simulink model "QPSK_NDATED_DDPED_R2021"  (R2021b)
settings: Solver=ode45  StartTime=0  StopTime=800*6  RelTol=1e-3  EnableMultiTasking=on
PreLoadFcn:
  | SNR=15;                          % Signal-to-noise ratio
  | T =  0.1;                          % Symbol period
  | Tc = T/10;                       % Carrier period
  | deltaf = (3/360)/T;;         % Frequency error
  | deltaT = 300e-6;             % Timing error
  | Tr = T*(1+deltaT);           % Receiver clock
  | alpha = 0.5;                     % Rolloff factor
  | b3 = [1/6 -1/2  1/2 -1/6];
  | b2 = [1/2 -1    1/2  0];
  | b1 = [1/3  1/2 -1    1/6];
  | b0 = [0    1    0    0];
  | warning off all
undefined symbols (not defined in the file or in its folder): dfilt, gcbh, rcfiltgaincompat
libraries: dspobslib x7, commfilt2 x4, dsparch4 x3, commchan3 x1, commdigbbndpm3 x1, commrandsrc2 x1
settings Model: SimulationMode=accelerator  Creator=professor  LastModifiedBy=14083
settings SolverCC: AlgebraicLoopSolver=TrustRegion
settings DataIOCC: LimitDataPoints=on  SaveFormat=Array  SignalLoggingSaveFormat=ModelDataLogs  ReturnWorkspaceOutputs=off
settings OptimizationCC: ExpressionDepthLimit=2147483647  InitFltsAndDblsToZero=on  LifeSpan=inf
settings DebuggingCC: AlgebraicLoopMsg=none  SaveWithParameterizedLinksMsg=none  UnderspecifiedInitializationDetection=Classic  MergeDetectMultiDrivingBlocksExec=none  SolverPrmCheckMsg=warning  MultiTaskDSMMsg=warning  MultiTaskCondExecSysMsg=none  FcnCallInpInsideContextMsg=warning  StateNameClashWarn=warning  SFUnexpectedBacktrackingDiag=warning  SFNoUnconditionalDefaultTransitionDiag=warning  SFExecutionAtInitializationDiag=none  SFMachineParentedDataDiag=warning  ArithmeticOperatorsInVariantConditions=warning
settings HardwareCC: ProdBitPerPointer=32  ProdBitPerSizeT=32  ProdBitPerPtrDiffT=32  ProdLargestAtomicFloat=None  ProdIntDivRoundTo=Undefined  ProdEndianess=Unspecified  ProdWordSize=32  ProdHWDeviceType=32-bit Generic
settings ModelReferenceCC: PropagateSignalLabelsOutOfModel=off
settings SFSimCC: SimUseLocalCustomCode=off  CustomCodeUndefinedFunction=UseInterfaceOnly
settings RTWCC: RTWUseLocalCustomCode=off
settings CodeAppCC: StateflowObjectComments=on
settings GRTTargetCC: TargetFcnLib=ansi_tfl_tmw.mat  TargetLangStandard=C89/C90 (ANSI)  CombineOutputUpdateFcns=off  GRTInterface=on
settings ConfigComp: CovMetricSettings=dw  CovSaveCumulativeToWorkspaceVar=on  CovSaveSingleToWorkspaceVar=on  CovExternalEMLEnable=off

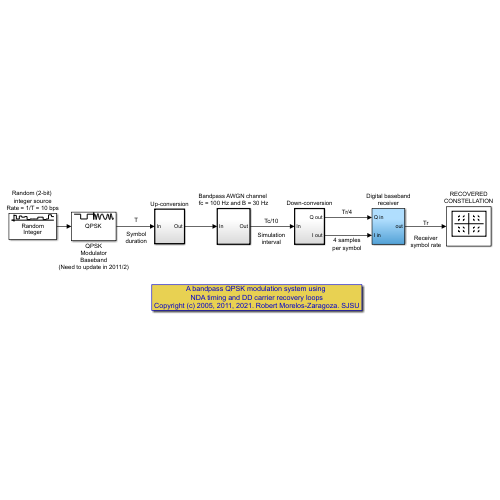
[thumbnail: Simulink's stored preview of the top-level diagram]
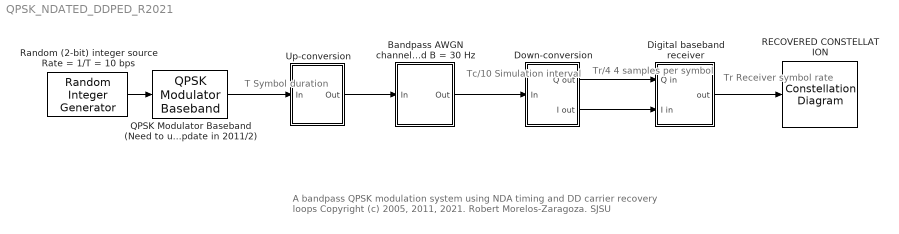
== system QPSK_NDATED_DDPED_R2021 ==
  note: A bandpass QPSK modulation system using
      | NDA timing and DD carrier recovery loops
      | Copyright (c) 2005, 2011, 2021. Robert Morelos-Zaragoza. SJSU
  note: Tc/10
      |
      | Simulation
      | interval
  note: T
      |
      | Symbol
      | duration
  note: Tr/4
      |
      |
      |
      | 4 samples
      | per symbol
  note: Tr
      |
      | Receiver
      | symbol rate
  Bandpass AWGN channel fc = 100 Hz and B = 30 Hz : Subsystem  TreatAsAtomicUnit=on
  Digital baseband receiver : Subsystem
  Down-conversion : Subsystem  TreatAsAtomicUnit=on
  QPSK Modulator Baseband (Need to update in 2011/2) : commdigbbndpm3/QPSK Modulator Baseband  InType=Integer  Enc=Gray  Ph=pi/4  outDtype=double  outWordLen=16  outUDDataType=sfix(16)  outFracLenMode=Best precision  outFracLen=15  outDataTypeStr=double  outLastDataTypeStr=double
  RECOVERED CONSTELLATION : ConstellationDiagram  Tag=ScatterPlot
  Random (2-bit) integer source Rate = 1/T = 10 bps : commrandsrc2/Random Integer Generator  mul=4  seed=15571  Ts=T  frameBased=off  sampPerFrame=1  orient=off  outDataType=double
      settings: SourceProductBaseCode=CM
  Up-conversion : Subsystem  TreatAsAtomicUnit=on
  wires:
  Bandpass AWGN channel fc = 100 Hz and B = 30 Hz/1(Out) -> Down-conversion/1(In)
  Down-conversion/1(Q out) -> Digital baseband receiver/1(Q in)
  Down-conversion/2(I out) -> Digital baseband receiver/2(I in)
  Digital baseband receiver/1(out) -> RECOVERED CONSTELLATION/1
  QPSK Modulator Baseband (Need to update in 2011/2)/1 -> Up-conversion/1(In)
  Random (2-bit) integer source Rate = 1/T = 10 bps/1 -> QPSK Modulator Baseband (Need to update in 2011/2)/1
  Up-conversion/1(Out) -> Bandpass AWGN channel fc = 100 Hz and B = 30 Hz/1(In)

== system QPSK_NDATED_DDPED_R2021/Bandpass AWGN channel fc = 100 Hz and B = 30 Hz ==
  note: Bandpass AWGN channel
      |
      | Robert Morelos-Zaragoza
      | San Jose State University
      | Copyright (c) 2005
  In : Inport
  AWGN Channel : commchan3/AWGN Channel  InputProcessing=Columns as channels (frame based)  seed=13357  noiseMode="Signal to noise ratio  (Eb/No)"  EbNodB=SNR  EsNodB=15  SNRdB=10  bitsPerSym=2  Ps=1  Tsym=T/4  variance=1
  "Channel Hc(f) fc=100, B=30" : dsparch4/Analog Filter Design  method=Chebyshev I  filttype=Bandpass  N=20  Wlo=2*pi*85  Whi=2*pi*115  Rp=0.5  Rs=30
  Tc/10 Simulation interval : ZeroOrderHold  SampleTime=Tc/10
  Out : Outport
  wires:
  "Channel Hc(f) fc=100, B=30"/1 -> Tc/10 Simulation interval/1
  AWGN Channel/1 -> Out/1
  In/1 -> "Channel Hc(f) fc=100, B=30"/1
  Tc/10 Simulation interval/1 -> AWGN Channel/1

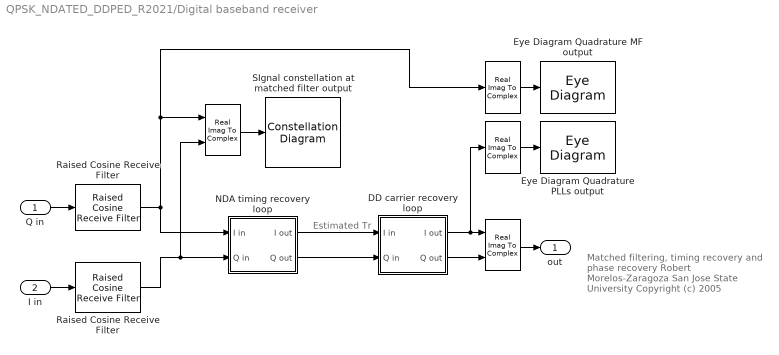
== system QPSK_NDATED_DDPED_R2021/Digital baseband receiver ==
  note: Estimated
      | Tr
  note: Matched filtering, timing recovery
      | and phase recovery
      |
      | Robert Morelos-Zaragoza
      | San Jose State University
      | Copyright (c) 2005
  Q in : Inport
  I in : Inport  Port=2
  " " : RealImagToComplex  Input=Real  SampleTime=Tr/4
  "    " : RealImagToComplex  SampleTime=Tr/4
  "       " : RealImagToComplex  Input=Real  SampleTime=Tr/4
  "           " : RealImagToComplex  SampleTime=Tr
  DD carrier recovery loop : Subsystem
  Eye Diagram Quadrature MF output : EyeDiagram  Tag=EyeDiagram
  Eye Diagram Quadrature PLLs output : EyeDiagram  Tag=EyeDiagram
  NDA timing recovery loop : Subsystem
  Raised Cosine Receive Filter : commfilt2/Raised Cosine Receive Filter  filtType=Square root  R=alpha  filtSpan=2*(4)  N=4  downFactor=1  downOffset=0  filterGain=(1/2)*rcfiltgaincompat(gcbh)  InputProcessing=Columns as channels (frame based)  RateOptions=Enforce single-rate processing  framing=Maintain input frame size  checkCoeff=off  variableName=rcRxFilt  currentFiltSpan=2*(4)  D=4  inputOffset=0  sampMode=Mute  saveAsFlag=0  rateMode=Downsampling  checkGain=User-specified  launchFVT=off  roundingMode=Floor  overflowMode=off  coeffDataTypeStr=Inherit: Same word length as input  coeffMin=[]  coeffMax=[]  coeffLastDataTypeStr=Inherit: Same word length as input  accumDataTypeStr=Inherit: Same as product output  accumLastDataTypeStr=Inherit: Same as product output  outputDataTypeStr=Inherit: Same as accumulator  outputMin=[]  outputMax=[]  outputLastDataTypeStr=Inherit: Same as accumulator
  "Raised Cosine Receive Filter " : commfilt2/Raised Cosine Receive Filter  filtType=Square root  R=alpha  filtSpan=2*(4)  N=4  downFactor=1  downOffset=0  filterGain=(1/2)*rcfiltgaincompat(gcbh)  InputProcessing=Columns as channels (frame based)  RateOptions=Enforce single-rate processing  framing=Maintain input frame size  checkCoeff=off  variableName=rcRxFilt1  currentFiltSpan=2*(4)  D=4  inputOffset=0  sampMode=Mute  saveAsFlag=0  rateMode=Downsampling  checkGain=User-specified  launchFVT=off  roundingMode=Floor  overflowMode=off  coeffDataTypeStr=Inherit: Same word length as input  coeffMin=[]  coeffMax=[]  coeffLastDataTypeStr=Inherit: Same word length as input  accumDataTypeStr=Inherit: Same as product output  accumLastDataTypeStr=Inherit: Same as product output  outputDataTypeStr=Inherit: Same as accumulator  outputMin=[]  outputMax=[]  outputLastDataTypeStr=Inherit: Same as accumulator
  SIgnal constellation at matched filter output : ConstellationDiagram  Tag=ScatterPlot
  out : Outport
  wires:
  Q in/1 -> Raised Cosine Receive Filter/1
  I in/1 -> "Raised Cosine Receive Filter "/1
  Raised Cosine Receive Filter/1 -> "    "/1, " "/1, NDA timing recovery loop/1(I in)
  "    "/1 -> SIgnal constellation at matched filter output/1
  DD carrier recovery loop/1(I out) -> "           "/1, "       "/1
  DD carrier recovery loop/2(Q out) -> "           "/2
  "           "/1 -> out/1
  NDA timing recovery loop/1(I out) -> DD carrier recovery loop/1(I in)
  NDA timing recovery loop/2(Q out) -> DD carrier recovery loop/2(Q in)
  " "/1 -> Eye Diagram Quadrature MF output/1
  "       "/1 -> Eye Diagram Quadrature PLLs output/1
  "Raised Cosine Receive Filter "/1 -> NDA timing recovery loop/2(Q in), "    "/2

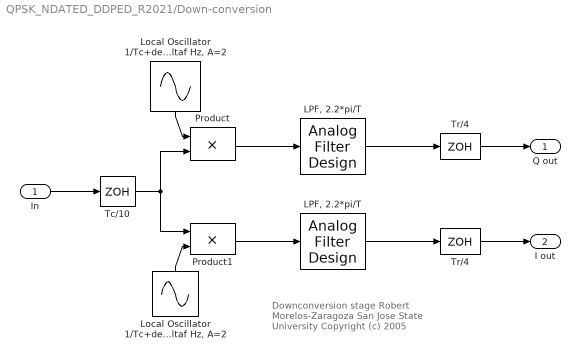
== system QPSK_NDATED_DDPED_R2021/Down-conversion ==
  note: Downconversion stage
      |
      | Robert Morelos-Zaragoza
      | San Jose State University
      | Copyright (c) 2005
  In : Inport
  " LPF, 2.2*pi/T " : dsparch4/Analog Filter Design  method=Butterworth  filttype=Lowpass  N=8  Wlo=2.2*pi/T  Whi=80  Rp=2  Rs=40
  "LPF, 2.2*pi/T" : dsparch4/Analog Filter Design  method=Butterworth  filttype=Lowpass  N=8  Wlo=2.2*pi/T  Whi=80  Rp=2  Rs=40
  "Local Oscillator 1/Tc+deltaf Hz, A=2 " : Sin  Amplitude=2  Frequency=2*pi/Tc+deltaf  SampleTime=Tc/10
  "Local Oscillator 1/Tc+deltaf Hz, A=2    " : Sin  Amplitude=2  Frequency=2*pi/Tc+deltaf  Phase=pi/2  SampleTime=Tc/10
  Product : Product  InputSameDT=on  SaturateOnIntegerOverflow=on  OutDataTypeStr=Inherit: Same as first input
  Product1 : Product  InputSameDT=on  SaturateOnIntegerOverflow=on  OutDataTypeStr=Inherit: Same as first input
  Tc/10 : ZeroOrderHold  SampleTime=Tc/10
  Tr/4 : ZeroOrderHold  SampleTime=Tr/4
  "Tr/4 " : ZeroOrderHold  SampleTime=Tr/4
  Q out : Outport
  I out : Outport  Port=2
  wires:
  "Local Oscillator 1/Tc+deltaf Hz, A=2    "/1 -> Product1/2
  "LPF, 2.2*pi/T"/1 -> Tr/4/1
  "Local Oscillator 1/Tc+deltaf Hz, A=2 "/1 -> Product/1
  Product/1 -> "LPF, 2.2*pi/T"/1
  " LPF, 2.2*pi/T "/1 -> "Tr/4 "/1
  Product1/1 -> " LPF, 2.2*pi/T "/1
  In/1 -> Tc/10/1
  Tr/4/1 -> Q out/1
  "Tr/4 "/1 -> I out/1
  Tc/10/1 -> Product/2, Product1/1

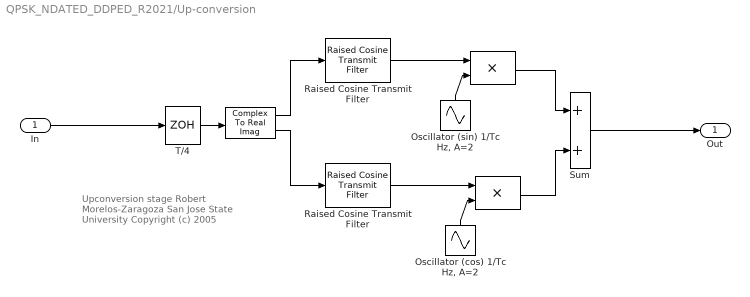
== system QPSK_NDATED_DDPED_R2021/Up-conversion ==
  note: Upconversion stage
      |
      | Robert Morelos-Zaragoza
      | San Jose State University
      | Copyright (c) 2005
  In : Inport
  " " : ComplexToRealImag
  "  " : Product  InputSameDT=on  SaturateOnIntegerOverflow=on  OutDataTypeStr=Inherit: Same as first input
  "   " : Product  InputSameDT=on  SaturateOnIntegerOverflow=on  OutDataTypeStr=Inherit: Same as first input
  "Oscillator (cos) 1/Tc Hz, A=2" : Sin  Amplitude=2  Frequency=2*pi/Tc  Phase=pi/2  SampleTime=0
  "Oscillator (sin) 1/Tc Hz, A=2 " : Sin  Amplitude=2  Frequency=2*pi/Tc  SampleTime=0
  Raised Cosine Transmit Filter : commfilt2/Raised Cosine Transmit Filter  filtType=Square root  R=alpha  filtSpan=2*(4)  N=4  filterGain=rcfiltgaincompat(gcbh)  RateOptions=Allow multirate processing  framing=Maintain input frame size  checkCoeff=off  variableName=rcTxFilt  checkGain=Normalized  sampMode=Mute  saveAsFlag=0  currentFiltSpan=2*(4)  D=4  launchFVT=off  roundingMode=Floor  overflowMode=off  coeffDataTypeStr=Inherit: Same word length as input  coeffMin=[]  coeffMax=[]  coeffLastDataTypeStr=Inherit: Same word length as input  outputDataTypeStr=Inherit: Same as accumulator  outputMin=[]  outputMax=[]  outputLastDataTypeStr=Inherit: Same as accumulator
  "Raised Cosine Transmit Filter " : commfilt2/Raised Cosine Transmit Filter  filtType=Square root  R=alpha  filtSpan=2*(4)  N=4  filterGain=rcfiltgaincompat(gcbh)  RateOptions=Allow multirate processing  framing=Maintain input frame size  checkCoeff=off  variableName=rcTxFilt1  checkGain=Normalized  sampMode=Mute  saveAsFlag=0  currentFiltSpan=2*(4)  D=4  launchFVT=off  roundingMode=Floor  overflowMode=off  coeffDataTypeStr=Inherit: Same word length as input  coeffMin=[]  coeffMax=[]  coeffLastDataTypeStr=Inherit: Same word length as input  outputDataTypeStr=Inherit: Same as accumulator  outputMin=[]  outputMax=[]  outputLastDataTypeStr=Inherit: Same as accumulator
  Sum : Sum  InputSameDT=on  SaturateOnIntegerOverflow=on  OutDataTypeStr=Inherit: Same as first input
  T/4 : ZeroOrderHold  SampleTime=T/4
  Out : Outport
  wires:
  T/4/1 -> " "/1
  In/1 -> T/4/1
  Raised Cosine Transmit Filter/1 -> "  "/1
  "Raised Cosine Transmit Filter "/1 -> "   "/1
  "Oscillator (sin) 1/Tc Hz, A=2 "/1 -> "  "/2
  "Oscillator (cos) 1/Tc Hz, A=2"/1 -> "   "/2
  "  "/1 -> Sum/1
  "   "/1 -> Sum/2
  Sum/1 -> Out/1
  " "/1 -> Raised Cosine Transmit Filter/1
  " "/2 -> "Raised Cosine Transmit Filter "/1

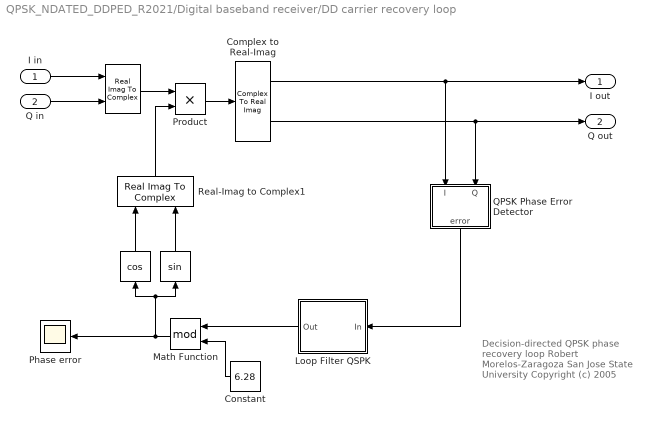
== system QPSK_NDATED_DDPED_R2021/Digital baseband receiver/DD carrier recovery loop ==
  note: Decision-directed QPSK
      | phase recovery loop
      |
      | Robert Morelos-Zaragoza
      | San Jose State University
      | Copyright (c) 2005
  I in : Inport
  Q in : Inport  Port=2
  " " : Trigonometry  OutputSignalType=real
  "   " : Trigonometry  Operator=cos  OutputSignalType=real
  "     " : RealImagToComplex  SampleTime=Tr
  "  QPSK Phase Error Detector" : Subsystem
  Complex to Real-Imag : ComplexToRealImag
  Constant : Constant  Value=6.28  SampleTime=Tr
  Loop Filter QSPK : Subsystem
  Math Function : Math  Operator=mod  SignedPower=on  OutputSignalType=real  SampleTime=Tr  SaturateOnIntegerOverflow=on
  Phase error : Scope
  Product : Product  InputSameDT=on  OutDataTypeStr=Inherit: Same as first input
  Real-Imag to Complex1 : RealImagToComplex
  I out : Outport
  Q out : Outport  Port=2
  wires:
  Real-Imag to Complex1/1 -> Product/2
  "   "/1 -> Real-Imag to Complex1/1
  " "/1 -> Real-Imag to Complex1/2
  Product/1 -> Complex to Real-Imag/1
  Complex to Real-Imag/1 -> I out/1, "  QPSK Phase Error Detector"/1(I)
  Complex to Real-Imag/2 -> Q out/1, "  QPSK Phase Error Detector"/2(Q)
  Loop Filter QSPK/1(Out) -> Math Function/1
  Constant/1 -> Math Function/2
  Math Function/1 -> " "/1, "   "/1, Phase error/1
  I in/1 -> "     "/1
  Q in/1 -> "     "/2
  "     "/1 -> Product/1
  "  QPSK Phase Error Detector"/1(error) -> Loop Filter QSPK/1(In)

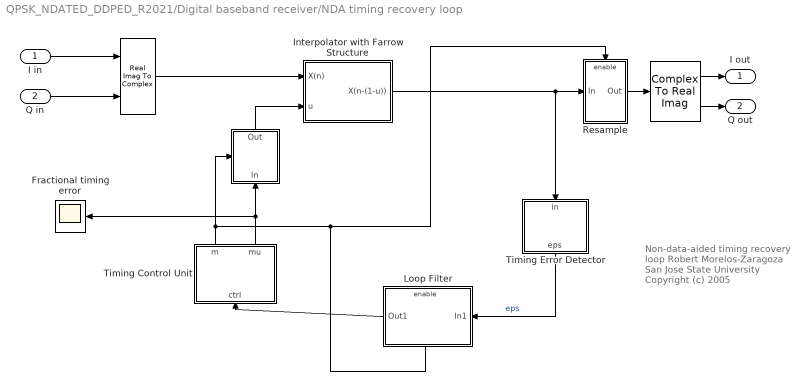
== system QPSK_NDATED_DDPED_R2021/Digital baseband receiver/NDA timing recovery loop ==
  note: Non-data-aided timing
      | recovery loop
      |
      | Robert Morelos-Zaragoza
      | San Jose State University
      | Copyright (c) 2005
  I in : Inport
  Q in : Inport  Port=2
  " " : ComplexToRealImag
  "     " : RealImagToComplex  SampleTime=Tr/4
  "         " : Subsystem  TreatAsAtomicUnit=on
  "  Timing Error Detector " : Subsystem
  Fractional timing error : Scope
  "Interpolator with Farrow Structure " : Subsystem
  "Loop Filter " : Subsystem  TreatAsAtomicUnit=on
  Resample : Subsystem  TreatAsAtomicUnit=on
  "Timing Control Unit   " : Subsystem
  I out : Outport
  Q out : Outport  Port=2
  wires:
  I in/1 -> "     "/1
  Q in/1 -> "     "/2
  "Interpolator with Farrow Structure "/1(X(n-(1-u))) -> Resample/1(In), "  Timing Error Detector "/1(in)
  "     "/1 -> "Interpolator with Farrow Structure "/1(X(n))
  "  Timing Error Detector "/1(eps) -> "Loop Filter "/1(In1)  "eps"
  " "/1 -> I out/1
  " "/2 -> Q out/1
  Resample/1(Out) -> " "/1
  "Loop Filter "/1(Out1) -> "Timing Control Unit   "/1(ctrl)
  "Timing Control Unit   "/2(mu) -> "         "/1(In), Fractional timing error/1
  "         "/1(Out) -> "Interpolator with Farrow Structure "/2(u)
  "Timing Control Unit   "/1(m) -> "         "/Enable, Resample/Enable, "Loop Filter "/Enable

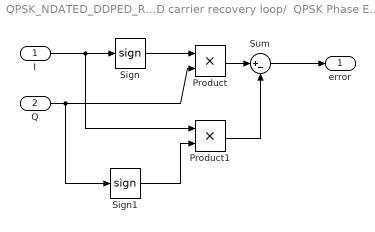
== system QPSK_NDATED_DDPED_R2021/Digital baseband receiver/DD carrier recovery loop/  QPSK Phase Error Detector ==
  I : Inport
  Q : Inport  Port=2
  Product : Product  InputSameDT=on  SaturateOnIntegerOverflow=on  SampleTime=Tr  OutDataTypeStr=Inherit: Same as first input
  Product1 : Product  InputSameDT=on  SaturateOnIntegerOverflow=on  SampleTime=Tr  OutDataTypeStr=Inherit: Same as first input
  Sign : Signum  SampleTime=Tr
  Sign1 : Signum  SampleTime=Tr
  Sum : Sum  Inputs=|+-  InputSameDT=on  SaturateOnIntegerOverflow=on  OutDataTypeStr=Inherit: Same as first input
  error : Outport
  wires:
  Sign/1 -> Product/1
  I/1 -> Sign/1, Product1/1
  Q/1 -> Product/2, Sign1/1
  Sign1/1 -> Product1/2
  Sum/1 -> error/1
  Product/1 -> Sum/1
  Product1/1 -> Sum/2

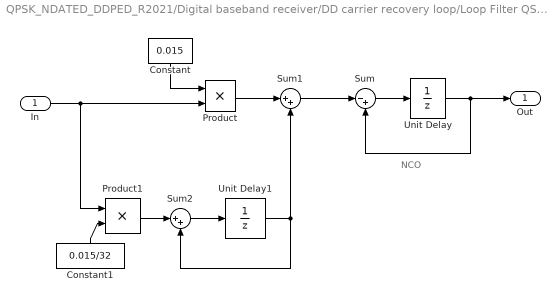
== system QPSK_NDATED_DDPED_R2021/Digital baseband receiver/DD carrier recovery loop/Loop Filter QSPK ==
  note: NCO
  In : Inport
  Constant : Constant  Value=0.015  SampleTime=Tr
  Constant1 : Constant  Value=0.015/32  SampleTime=Tr
  Product : Product  InputSameDT=on  SaturateOnIntegerOverflow=on  SampleTime=Tr  OutDataTypeStr=Inherit: Same as first input
  Product1 : Product  InputSameDT=on  SaturateOnIntegerOverflow=on  SampleTime=Tr  OutDataTypeStr=Inherit: Same as first input
  Sum : Sum  Inputs=|-+  InputSameDT=on  SaturateOnIntegerOverflow=on  OutDataTypeStr=Inherit: Same as first input
  Sum1 : Sum  Inputs=|++  InputSameDT=on  SaturateOnIntegerOverflow=on  OutDataTypeStr=Inherit: Same as first input
  Sum2 : Sum  Inputs=|++  InputSameDT=on  SaturateOnIntegerOverflow=on  OutDataTypeStr=Inherit: Same as first input
  Unit Delay : UnitDelay  SampleTime=Tr  HasFrameUpgradeWarning=on
  Unit Delay1 : UnitDelay  SampleTime=Tr  HasFrameUpgradeWarning=on
  Out : Outport
  wires:
  Product/1 -> Sum1/1
  Constant1/1 -> Product1/2
  Sum/1 -> Unit Delay/1
  Unit Delay/1 -> Out/1, Sum/2
  Constant/1 -> Product/1
  In/1 -> Product/2, Product1/1
  Product1/1 -> Sum2/1
  Sum2/1 -> Unit Delay1/1
  Unit Delay1/1 -> Sum1/2, Sum2/2
  Sum1/1 -> Sum/1

== system QPSK_NDATED_DDPED_R2021/Digital baseband receiver/NDA timing recovery loop/          ==
  In : Inport
  Enable : EnablePort
  Out : Outport
  wires:
  In/1 -> Out/1

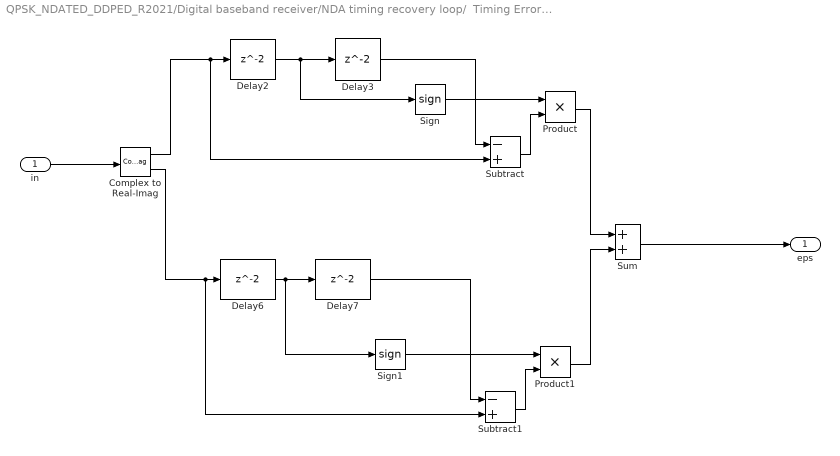
== system QPSK_NDATED_DDPED_R2021/Digital baseband receiver/NDA timing recovery loop/  Timing Error Detector  ==
  in : Inport
  Complex to Real-Imag : ComplexToRealImag
  Delay{2..3,6..7} (4 alike) : Delay  InitialCondition=0
  Product : Product  RndMeth=Zero
  Product1 : Product  RndMeth=Zero
  Sign : Signum
  Sign1 : Signum
  Subtract : Sum  Inputs=-+
  Subtract1 : Sum  Inputs=-+
  Sum : Sum
  eps : Outport
  wires:
  Delay3/1 -> Subtract/1
  Delay7/1 -> Subtract1/1
  in/1 -> Complex to Real-Imag/1
  Complex to Real-Imag/1 -> Delay2/1, Subtract/2
  Complex to Real-Imag/2 -> Delay6/1, Subtract1/2
  Sum/1 -> eps/1
  Subtract1/1 -> Product1/2
  Product1/1 -> Sum/2
  Subtract/1 -> Product/2
  Product/1 -> Sum/1
  Delay2/1 -> Delay3/1, Sign/1
  Delay6/1 -> Delay7/1, Sign1/1
  Sign/1 -> Product/1
  Sign1/1 -> Product1/1

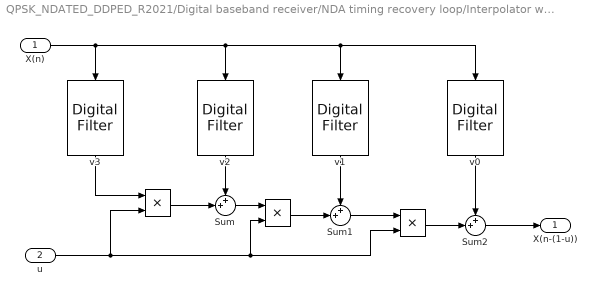
== system QPSK_NDATED_DDPED_R2021/Digital baseband receiver/NDA timing recovery loop/Interpolator with Farrow Structure  ==
  X(n) : Inport
  u : Inport  Port=2
  " " : Product  SaturateOnIntegerOverflow=on  OutDataTypeStr=Inherit: Same as first input
  "  " : Product  SaturateOnIntegerOverflow=on  OutDataTypeStr=Inherit: Same as first input
  "   " : Product  SaturateOnIntegerOverflow=on  OutDataTypeStr=Inherit: Same as first input
  Sum : Sum  Inputs=++|  SaturateOnIntegerOverflow=on
  Sum1 : Sum  Inputs=++|  SaturateOnIntegerOverflow=on
  Sum2 : Sum  Inputs=++|  SaturateOnIntegerOverflow=on
  v0 : dspobslib/Digital Filter  TypePopup=FIR (all zeros)  IIRFiltStruct=Direct form II transposed  AllPoleFiltStruct=Direct form  FIRFiltStruct=Direct form  CoeffSource=Specify via dialog  NumCoeffs=b0  DenCoeffs=[1 0.1]  BiQuadCoeffs=[1 0.3 0.4 1 0.1 0.2]  LatticeCoeffs=[0.2 0.4]  denIgnore=on  FiltPerSampPopup=One filter per frame  IC=0  ICnum=0  ICden=0  roundingMode=Floor  overflowMode=off  ScaleValues=1  scaleValueFracLength=14  stageInFracLength=15  stageOutFracLength=15  FilterSource=Specify via dialog  dfiltObjectName=dfilt.dffir([1 2 1])  InputProcessing=Inherited (this choice will be removed - see release notes)
      settings: SourceProductBaseCode=DS
  v1 : dspobslib/Digital Filter  TypePopup=FIR (all zeros)  IIRFiltStruct=Direct form II transposed  AllPoleFiltStruct=Direct form  FIRFiltStruct=Direct form  CoeffSource=Specify via dialog  NumCoeffs=b1  DenCoeffs=[1 0.1]  BiQuadCoeffs=[1 0.3 0.4 1 0.1 0.2]  LatticeCoeffs=[0.2 0.4]  denIgnore=on  FiltPerSampPopup=One filter per frame  IC=0  ICnum=0  ICden=0  roundingMode=Floor  overflowMode=off  ScaleValues=1  scaleValueFracLength=14  stageInFracLength=15  stageOutFracLength=15  FilterSource=Specify via dialog  dfiltObjectName=dfilt.dffir([1 2 1])  InputProcessing=Inherited (this choice will be removed - see release notes)
      settings: SourceProductBaseCode=DS
  v2 : dspobslib/Digital Filter  TypePopup=FIR (all zeros)  IIRFiltStruct=Direct form II transposed  AllPoleFiltStruct=Direct form  FIRFiltStruct=Direct form  CoeffSource=Specify via dialog  NumCoeffs=b2  DenCoeffs=[1 0.1]  BiQuadCoeffs=[1 0.3 0.4 1 0.1 0.2]  LatticeCoeffs=[0.2 0.4]  denIgnore=on  FiltPerSampPopup=One filter per frame  IC=0  ICnum=0  ICden=0  roundingMode=Floor  overflowMode=off  ScaleValues=1  scaleValueFracLength=14  stageInFracLength=15  stageOutFracLength=15  FilterSource=Specify via dialog  dfiltObjectName=dfilt.dffir([1 2 1])  InputProcessing=Inherited (this choice will be removed - see release notes)
      settings: SourceProductBaseCode=DS
  v3 : dspobslib/Digital Filter  TypePopup=FIR (all zeros)  IIRFiltStruct=Direct form II transposed  AllPoleFiltStruct=Direct form  FIRFiltStruct=Direct form  CoeffSource=Specify via dialog  NumCoeffs=b3  DenCoeffs=[1 0.1]  BiQuadCoeffs=[1 0.3 0.4 1 0.1 0.2]  LatticeCoeffs=[0.2 0.4]  denIgnore=on  FiltPerSampPopup=One filter per frame  IC=0  ICnum=0  ICden=0  roundingMode=Floor  overflowMode=off  ScaleValues=1  scaleValueFracLength=14  stageInFracLength=15  stageOutFracLength=15  FilterSource=Specify via dialog  dfiltObjectName=dfilt.dffir([1 2 1])  InputProcessing=Inherited (this choice will be removed - see release notes)
      settings: SourceProductBaseCode=DS
  X(n-(1-u)) : Outport
  wires:
  Sum2/1 -> X(n-(1-u))/1
  u/1 -> "   "/2, "  "/2, " "/2
  X(n)/1 -> v3/1, v2/1, v1/1, v0/1
  v0/1 -> Sum2/1
  v1/1 -> Sum1/1
  v2/1 -> Sum/1
  v3/1 -> " "/1
  " "/1 -> Sum/2
  Sum/1 -> "  "/1
  "  "/1 -> Sum1/2
  Sum1/1 -> "   "/1
  "   "/1 -> Sum2/2

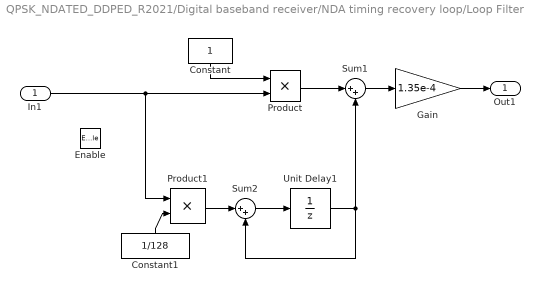
== system QPSK_NDATED_DDPED_R2021/Digital baseband receiver/NDA timing recovery loop/Loop Filter  ==
  In1 : Inport
  Enable : EnablePort
  Constant : Constant  SampleTime=Tr/4
  Constant1 : Constant  Value=1/128  SampleTime=Tr/4
  Gain : Gain  Gain=1.35e-4
  Product : Product  InputSameDT=on  SaturateOnIntegerOverflow=on  OutDataTypeStr=Inherit: Same as first input
  Product1 : Product  InputSameDT=on  SaturateOnIntegerOverflow=on  OutDataTypeStr=Inherit: Same as first input
  Sum1 : Sum  Inputs=|++  InputSameDT=on  SaturateOnIntegerOverflow=on  OutDataTypeStr=Inherit: Same as first input
  Sum2 : Sum  Inputs=|++  InputSameDT=on  SaturateOnIntegerOverflow=on  OutDataTypeStr=Inherit: Same as first input
  Unit Delay1 : UnitDelay  SampleTime=-1  HasFrameUpgradeWarning=on
  Out1 : Outport
  wires:
  Product/1 -> Sum1/1
  Constant1/1 -> Product1/2
  Constant/1 -> Product/1
  In1/1 -> Product/2, Product1/1
  Product1/1 -> Sum2/1
  Sum2/1 -> Unit Delay1/1
  Unit Delay1/1 -> Sum1/2, Sum2/2
  Sum1/1 -> Gain/1
  Gain/1 -> Out1/1

== system QPSK_NDATED_DDPED_R2021/Digital baseband receiver/NDA timing recovery loop/Resample ==
  In : Inport
  Enable : EnablePort
  Out : Outport
  wires:
  In/1 -> Out/1

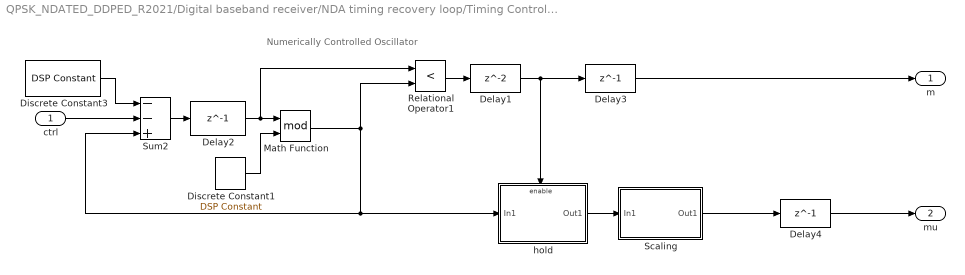
== system QPSK_NDATED_DDPED_R2021/Digital baseband receiver/NDA timing recovery loop/Timing Control Unit    ==
  note: Numerically Controlled Oscillator
  ctrl : Inport
  Delay1 : Delay  InitialCondition=0
  Delay2 : Delay  DelayLength=1  InitialCondition=0
  Delay3 : Delay  DelayLength=1  InitialCondition=0
  Delay4 : Delay  DelayLength=1  InitialCondition=0
  Discrete Constant1 : dspobslib/DSP Constant  Value=1  SampleMode=Discrete  discreteOutput=Sample-based (interpret vectors as 1-D)  continuousOutput=Sample-based  sampTime=Tr/4  framePeriod=Tr/4  dataType=Inherit via back propagation  isSigned=on  wordLen=16  udDataType=sfix(16)  fracBitsMode=Best precision  numFracBits=15  InterpretAs1D=on  Ts=Tr/4  FramebasedOutput=off
      settings: SourceProductBaseCode=DS  additionalParams=on
  Discrete Constant3 : dspobslib/DSP Constant  Value=1/4  SampleMode=Discrete  discreteOutput=Sample-based (interpret vectors as 1-D)  continuousOutput=Sample-based  sampTime=Tr/4  framePeriod=Tr/4  dataType=Inherit via back propagation  isSigned=on  wordLen=16  udDataType=sfix(16)  fracBitsMode=Best precision  numFracBits=15  InterpretAs1D=on  Ts=Tr/4  FramebasedOutput=off
      settings: SourceProductBaseCode=DS  additionalParams=on
  Math Function : Math  Operator=mod  SignedPower=on  SampleTime=Tr/4  SaturateOnIntegerOverflow=on
  Relational Operator1 : RelationalOperator  Operator=<  OutDataTypeStr=boolean  SampleTime=Tr/4  RndMeth=Nearest
  Scaling : Subsystem
  Sum2 : Sum  Inputs=--+  InputSameDT=on  SaturateOnIntegerOverflow=on  SampleTime=Tr/4  OutDataTypeStr=Inherit: Same as first input
  hold : Subsystem  TreatAsAtomicUnit=on
  m : Outport
  mu : Outport  Port=2
  wires:
  Delay2/1 -> Math Function/1, Relational Operator1/1
  Discrete Constant1/1 -> Math Function/2
  Sum2/1 -> Delay2/1
  ctrl/1 -> Sum2/2
  Math Function/1 -> Relational Operator1/2, hold/1(In1), Sum2/3
  Relational Operator1/1 -> Delay1/1
  hold/1(Out1) -> Scaling/1(In1)
  Discrete Constant3/1 -> Sum2/1
  Delay3/1 -> m/1
  Scaling/1(Out1) -> Delay4/1
  Delay4/1 -> mu/1
  Delay1/1 -> hold/Enable, Delay3/1

== system QPSK_NDATED_DDPED_R2021/Digital baseband receiver/NDA timing recovery loop/Timing Control Unit   /Scaling ==
  In1 : Inport
  Add : Sum
  Discrete Constant1 : dspobslib/DSP Constant  Value=1  SampleMode=Discrete  discreteOutput=Sample-based (interpret vectors as 1-D)  continuousOutput=Sample-based  sampTime=Tr/4  framePeriod=Tr/4  dataType=Inherit via back propagation  isSigned=on  wordLen=16  udDataType=sfix(16)  fracBitsMode=Best precision  numFracBits=15  InterpretAs1D=on  Ts=Tr/4  FramebasedOutput=off
      settings: SourceProductBaseCode=DS  additionalParams=on
  Gain2 : Gain  Gain=4
  Math Function : Math  Operator=mod  SignedPower=on  SaturateOnIntegerOverflow=on
  k5 : Constant  Value=-2  SampleTime=Tr/4
  Out1 : Outport
  wires:
  In1/1 -> Gain2/1
  k5/1 -> Add/2
  Gain2/1 -> Add/1
  Add/1 -> Math Function/1
  Math Function/1 -> Out1/1
  Discrete Constant1/1 -> Math Function/2

== system QPSK_NDATED_DDPED_R2021/Digital baseband receiver/NDA timing recovery loop/Timing Control Unit   /hold ==
  In1 : Inport
  Enable : EnablePort
  Out1 : Outport
  wires:
  In1/1 -> Out1/1
